simulink model "model5_2022b_localconn"  (R2022b)
settings: Solver=VariableStepAuto  StartTime=0.0  StopTime=10.0  RelTol=1e-3
values from neighbouring files (symbols this model uses):
  eps_local = 50    [init5.m]
  obj1 = [60, 45]    [init5.m]
  obj2 = [30, 25]    [init5.m]
  thr = 5    [init5.m]
undefined symbols (not defined in the file or in its folder): K1, K2, K3, K4, K5, X01, X02, X03, X04, X05, X1d, X1d_dot, X2d, X2d_dot, X3d, X3d_dot, X4d, X4d_dot, X5d, X5d_dot
libraries: slctrlblks x1
settings Model: Creator=dorec  LastModifiedBy=dorec

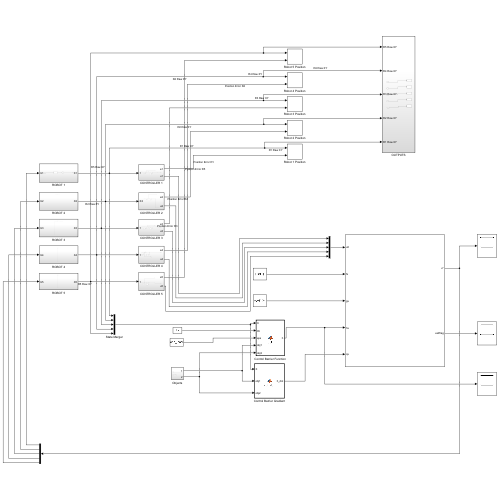
[thumbnail: Simulink's stored preview of the top-level diagram]
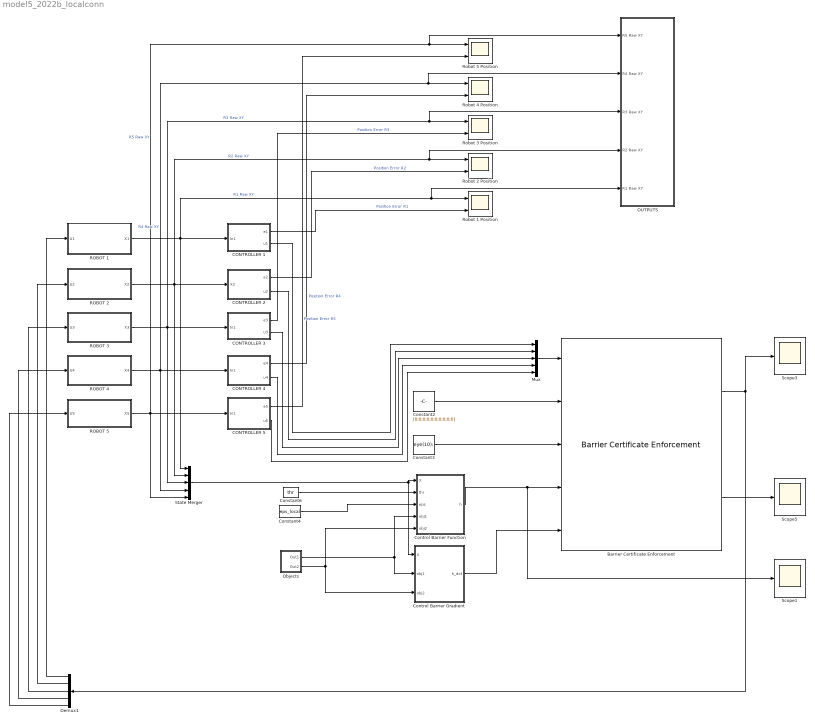
== system model5_2022b_localconn ==
  Barrier Certificate Enforcement : slctrlblks/Barrier Certificate Enforcement  nx=10  nu=10  nc=30  gamma=10  beta=1  external_umax=off  external_umin=off  Ts=0.1  maxiter=200  tol=1e-6  output_exitflag=on
      settings: LibrarySourceBlock=slctrlblks/Constraint Control/Barrier Certificate Enforcement
  CONTROLLER 1 : Subsystem
  CONTROLLER 2 : Subsystem
  CONTROLLER 3 : Subsystem
  CONTROLLER 4 : Subsystem
  CONTROLLER 5 : Subsystem
  Constant2 : Constant  Value=[0;0;0;0;0;0;0;0;0;0]
  Constant3 : Constant  Value=eye(10);
  Constant4 : Constant  Value=eps_local
  Constant6 : Constant  Value=thr
  Control Barrier Function : MATLAB Function  TreatAsAtomicUnit=on
  Control Barrier Gradient : MATLAB Function  TreatAsAtomicUnit=on
  Demux1 : Demux  Outputs=5
  Mux : Mux  Inputs=5
  OUTPUTS : Subsystem
  Objects : Subsystem
  ROBOT 1 : Subsystem
  ROBOT 2 : Subsystem
  ROBOT 3 : Subsystem
  ROBOT 4 : Subsystem
  ROBOT 5 : Subsystem
  Robot 1 Position : Scope  NumInputPorts=2
  Robot 2 Position : Scope  NumInputPorts=2
  Robot 3 Position : Scope  NumInputPorts=2
  Robot 4 Position : Scope  NumInputPorts=2
  Robot 5 Position : Scope  NumInputPorts=2
  Scope1 : Scope
  Scope3 : Scope
  Scope5 : Scope
  State Merger : Mux  Inputs=5
  wires:
  Control Barrier Function/1(h) -> Scope1/1, Barrier Certificate Enforcement/4
  Constant3/1 -> Barrier Certificate Enforcement/3
  Constant2/1 -> Barrier Certificate Enforcement/2
  Barrier Certificate Enforcement/1 -> Scope3/1, Demux1/1
  Mux/1 -> Barrier Certificate Enforcement/1
  Constant6/1 -> Control Barrier Function/2(thr)
  State Merger/1 -> Control Barrier Gradient/1(X), Control Barrier Function/1(X)
  Control Barrier Gradient/1(h_dot) -> Barrier Certificate Enforcement/5
  Barrier Certificate Enforcement/2 -> Scope5/1
  ROBOT 1/1(X1) -> OUTPUTS/5(R1 Raw XY), Robot 1 Position/1, CONTROLLER 1/1(In1), State Merger/1  "R1 Raw XY"
  Demux1/1 -> ROBOT 1/1(U1)
  CONTROLLER 1/2(u1) -> Mux/1
  ROBOT 2/1(X2) -> CONTROLLER 2/1(X2), OUTPUTS/4(R2 Raw XY), Robot 2 Position/1, State Merger/2  "R2 Raw XY"
  Demux1/2 -> ROBOT 2/1(U2)
  CONTROLLER 2/2(u2) -> Mux/2
  ROBOT 3/1(X3) -> OUTPUTS/3(R3 Raw XY), Robot 3 Position/1, CONTROLLER 3/1(In1), State Merger/3  "R3 Raw XY"
  Demux1/3 -> ROBOT 3/1(U3)
  CONTROLLER 3/1(e3) -> Robot 3 Position/2  "Position Error R3"
  CONTROLLER 3/2(u3) -> Mux/3
  ROBOT 4/1(X4) -> CONTROLLER 4/1(In1), OUTPUTS/2(R4 Raw XY), Robot 4 Position/1, State Merger/4  "R4 Raw XY"
  Demux1/4 -> ROBOT 4/1(U4)
  CONTROLLER 4/1(e4) -> Robot 4 Position/2  "Position Error R4"
  CONTROLLER 4/2(u4) -> Mux/4
  ROBOT 5/1(X5) -> OUTPUTS/1(R5 Raw XY), Robot 5 Position/1, CONTROLLER 5/1(In1), State Merger/5  "R5 Raw XY"
  Demux1/5 -> ROBOT 5/1(U5)
  CONTROLLER 5/2(u5) -> Mux/5
  CONTROLLER 5/1(e5) -> Robot 5 Position/2  "Position Error R5"
  CONTROLLER 1/1(e1) -> Robot 1 Position/2  "Position Error R1"
  CONTROLLER 2/1(e2) -> Robot 2 Position/2  "Position Error R2"
  Objects/2(Out2) -> Control Barrier Function/5(obj2), Control Barrier Gradient/3(obj2)
  Objects/1(Out1) -> Control Barrier Function/4(obj1), Control Barrier Gradient/2(obj1)
  Constant4/1 -> Control Barrier Function/3(eps)

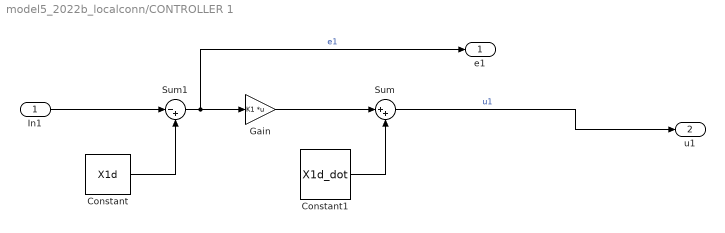
== system model5_2022b_localconn/CONTROLLER 1 ==
  In1 : Inport
  Constant : Constant  Value=X1d
  Constant1 : Constant  Value=X1d_dot
  Gain : Gain  Gain=K1  Multiplication=Matrix(K*u)
  Sum : Sum  Inputs=|++
  Sum1 : Sum  Inputs=|-+
  e1 : Outport
  u1 : Outport  Port=2
  wires:
  Constant/1 -> Sum1/2
  Constant1/1 -> Sum/2
  Sum/1 -> u1/1  "u1"
  Sum1/1 -> e1/1, Gain/1  "e1"
  In1/1 -> Sum1/1
  Gain/1 -> Sum/1

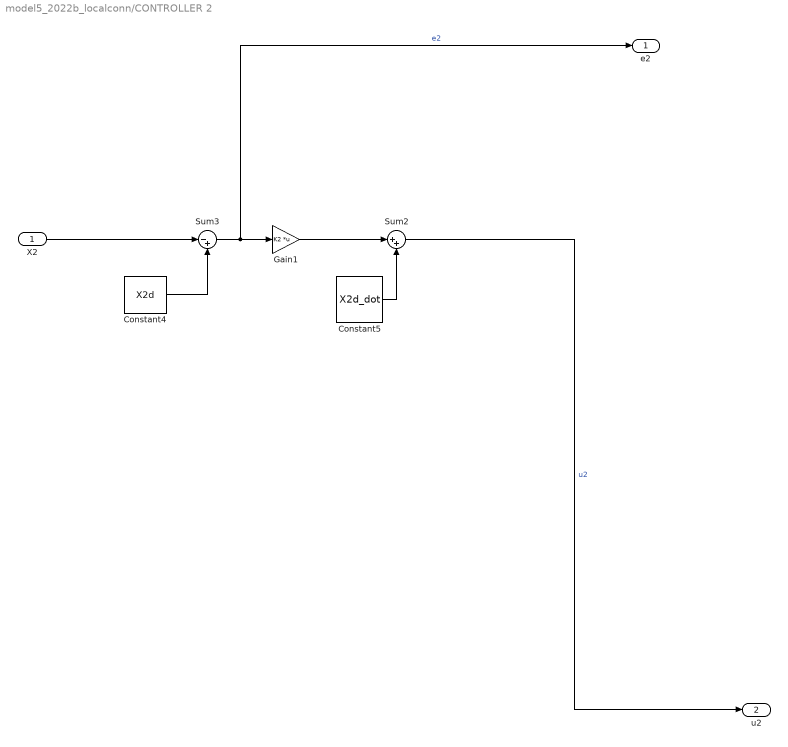
== system model5_2022b_localconn/CONTROLLER 2 ==
  X2 : Inport
  Constant4 : Constant  Value=X2d
  Constant5 : Constant  Value=X2d_dot
  Gain1 : Gain  Gain=K2  Multiplication=Matrix(K*u)
  Sum2 : Sum  Inputs=|++
  Sum3 : Sum  Inputs=|-+
  e2 : Outport
  u2 : Outport  Port=2
  wires:
  Constant4/1 -> Sum3/2
  Constant5/1 -> Sum2/2
  Sum3/1 -> e2/1, Gain1/1  "e2"
  Gain1/1 -> Sum2/1
  Sum2/1 -> u2/1  "u2"
  X2/1 -> Sum3/1

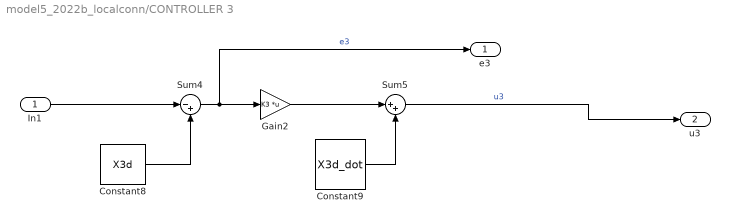
== system model5_2022b_localconn/CONTROLLER 3 ==
  In1 : Inport
  Constant8 : Constant  Value=X3d
  Constant9 : Constant  Value=X3d_dot
  Gain2 : Gain  Gain=K3  Multiplication=Matrix(K*u)
  Sum4 : Sum  Inputs=|-+
  Sum5 : Sum  Inputs=|++
  e3 : Outport
  u3 : Outport  Port=2
  wires:
  Constant9/1 -> Sum5/2
  Gain2/1 -> Sum5/1
  Sum4/1 -> e3/1, Gain2/1  "e3"
  Constant8/1 -> Sum4/2
  Sum5/1 -> u3/1  "u3"
  In1/1 -> Sum4/1

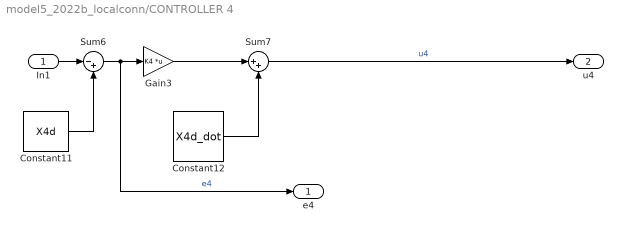
== system model5_2022b_localconn/CONTROLLER 4 ==
  In1 : Inport
  Constant11 : Constant  Value=X4d
  Constant12 : Constant  Value=X4d_dot
  Gain3 : Gain  Gain=K4  Multiplication=Matrix(K*u)
  Sum6 : Sum  Inputs=|-+
  Sum7 : Sum  Inputs=|++
  e4 : Outport
  u4 : Outport  Port=2
  wires:
  Sum6/1 -> e4/1, Gain3/1  "e4"
  Gain3/1 -> Sum7/1
  Constant11/1 -> Sum6/2
  Constant12/1 -> Sum7/2
  Sum7/1 -> u4/1  "u4"
  In1/1 -> Sum6/1

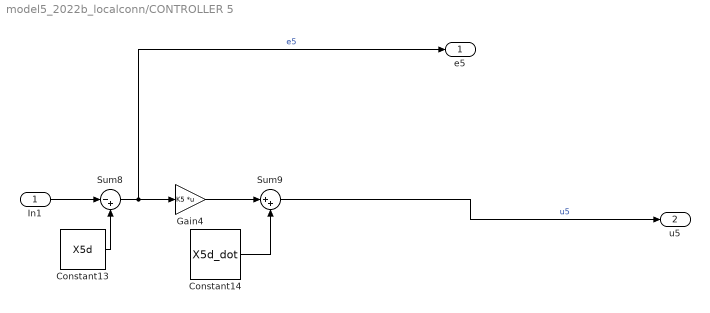
== system model5_2022b_localconn/CONTROLLER 5 ==
  In1 : Inport
  Constant13 : Constant  Value=X5d
  Constant14 : Constant  Value=X5d_dot
  Gain4 : Gain  Gain=K5  Multiplication=Matrix(K*u)
  Sum8 : Sum  Inputs=|-+
  Sum9 : Sum  Inputs=|++
  e5 : Outport
  u5 : Outport  Port=2
  wires:
  Sum8/1 -> e5/1, Gain4/1  "e5"
  Constant13/1 -> Sum8/2
  Gain4/1 -> Sum9/1
  In1/1 -> Sum8/1
  Constant14/1 -> Sum9/2
  Sum9/1 -> u5/1  "u5"

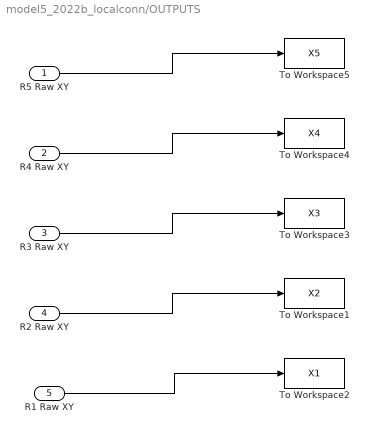
== system model5_2022b_localconn/OUTPUTS ==
  R5 Raw XY : Inport
  R4 Raw XY : Inport  Port=2
  R3 Raw XY : Inport  Port=3
  R2 Raw XY : Inport  Port=4
  R1 Raw XY : Inport  Port=5
  To Workspace1 : ToWorkspace  VariableName=X2  SaveFormat=Timeseries  SampleTime=-1
  To Workspace2 : ToWorkspace  VariableName=X1  SaveFormat=Timeseries  SampleTime=-1
  To Workspace3 : ToWorkspace  VariableName=X3  SaveFormat=Timeseries  SampleTime=-1
  To Workspace4 : ToWorkspace  VariableName=X4  SaveFormat=Timeseries  SampleTime=-1
  To Workspace5 : ToWorkspace  VariableName=X5  SaveFormat=Timeseries  SampleTime=-1
  wires:
  R5 Raw XY/1 -> To Workspace5/1
  R2 Raw XY/1 -> To Workspace1/1
  R1 Raw XY/1 -> To Workspace2/1
  R3 Raw XY/1 -> To Workspace3/1
  R4 Raw XY/1 -> To Workspace4/1

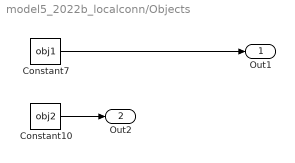
== system model5_2022b_localconn/Objects ==
  Constant10 : Constant  Value=obj2
  Constant7 : Constant  Value=obj1
  Out1 : Outport
  Out2 : Outport  Port=2
  wires:
  Constant10/1 -> Out2/1
  Constant7/1 -> Out1/1

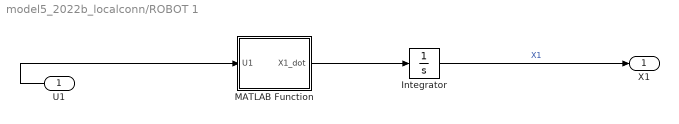
== system model5_2022b_localconn/ROBOT 1 ==
  U1 : Inport
  Integrator : Integrator  InitialCondition=X01
  MATLAB Function : MATLAB Function  TreatAsAtomicUnit=on
  X1 : Outport
  wires:
  MATLAB Function/1(X1_dot) -> Integrator/1
  Integrator/1 -> X1/1  "X1"
  U1/1 -> MATLAB Function/1(U1)

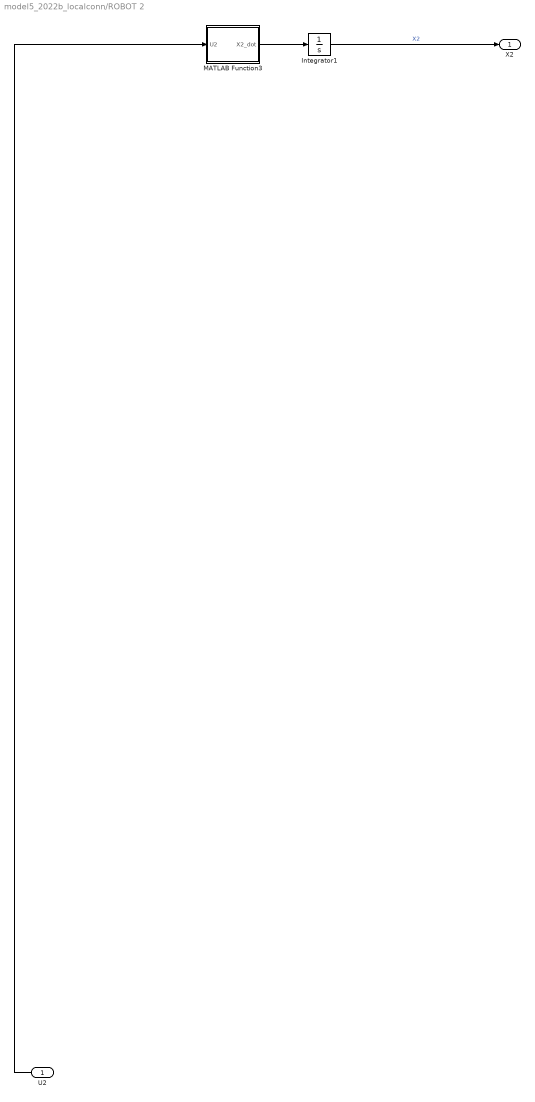
== system model5_2022b_localconn/ROBOT 2 ==
  U2 : Inport
  Integrator1 : Integrator  InitialCondition=X02
  MATLAB Function3 : MATLAB Function  TreatAsAtomicUnit=on
  X2 : Outport
  wires:
  MATLAB Function3/1(X2_dot) -> Integrator1/1
  U2/1 -> MATLAB Function3/1(U2)
  Integrator1/1 -> X2/1  "X2"

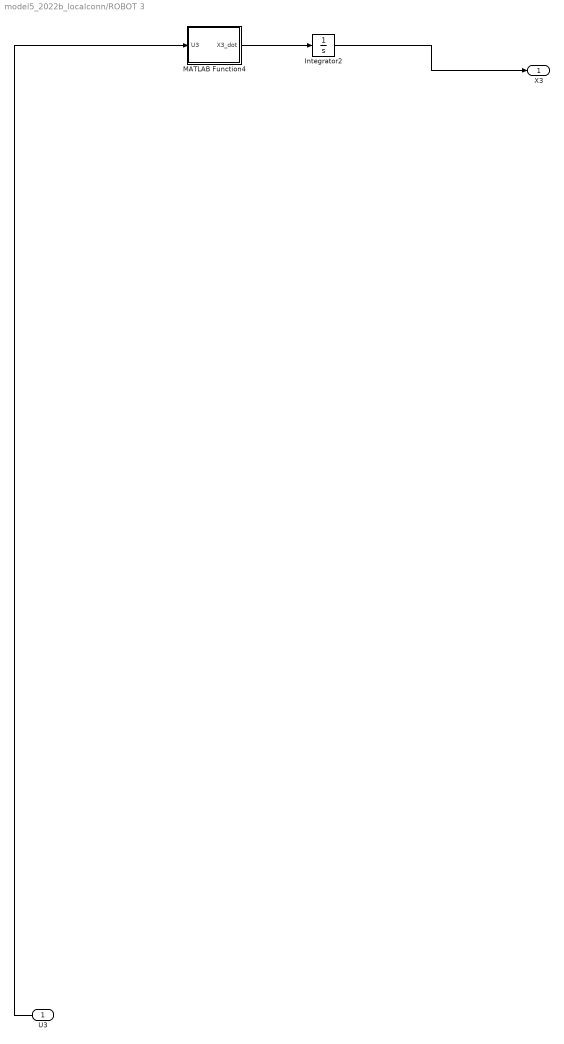
== system model5_2022b_localconn/ROBOT 3 ==
  U3 : Inport
  Integrator2 : Integrator  InitialCondition=X03
  MATLAB Function4 : MATLAB Function  TreatAsAtomicUnit=on
  X3 : Outport
  wires:
  U3/1 -> MATLAB Function4/1(U3)
  MATLAB Function4/1(X3_dot) -> Integrator2/1
  Integrator2/1 -> X3/1

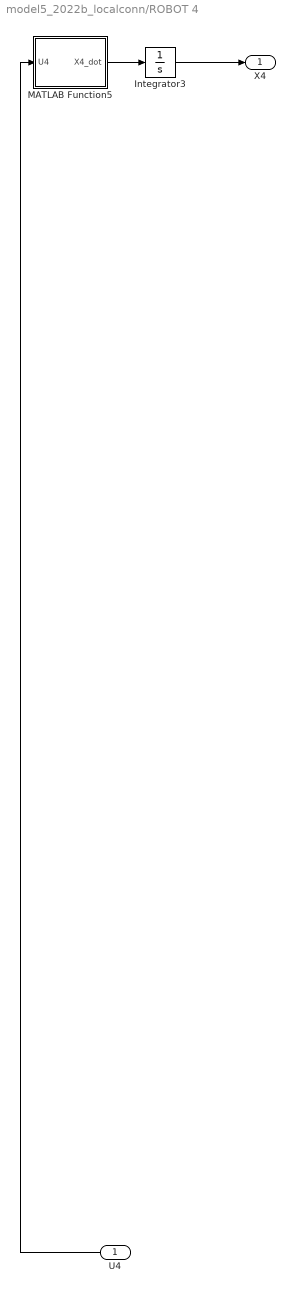
== system model5_2022b_localconn/ROBOT 4 ==
  U4 : Inport
  Integrator3 : Integrator  InitialCondition=X04
  MATLAB Function5 : MATLAB Function  TreatAsAtomicUnit=on
  X4 : Outport
  wires:
  MATLAB Function5/1(X4_dot) -> Integrator3/1
  U4/1 -> MATLAB Function5/1(U4)
  Integrator3/1 -> X4/1

== system model5_2022b_localconn/ROBOT 5 ==
  U5 : Inport
  Integrator4 : Integrator  InitialCondition=X05
  MATLAB Function6 : MATLAB Function  TreatAsAtomicUnit=on
  X5 : Outport
  wires:
  U5/1 -> MATLAB Function6/1(U5)
  MATLAB Function6/1(X5_dot) -> Integrator4/1
  Integrator4/1 -> X5/1

== matlab function model5_2022b_localconn/Control Barrier Function ==
  data: X input; thr input; eps input; h output; obj1 input; obj2 input
function h = cbf(X, thr, eps, obj1, obj2)

    %RESHAPES the vector from the mux (not stacked)
    Nvectors=numel(X)/2;
    X=reshape(X,2,Nvectors);
    
    %Extracts components col by col
    X1 = X(:,1);  
    X2 = X(:,2); 
    X3 = X(:,3);  
    X4 = X(:,4);  
    X5 = X(:,5);  

    h12 = norm(X1 - X2) - thr;
    h13 = norm(X1 - X3) - thr;
    h14 = norm(X1 - X4) - thr;
    h15 = norm(X1 - X5) - thr;

    h23 = norm(X2 - X3) - thr;
    h24 = norm(X2 - X4) - thr;
    h25 = norm(X2 - X5) - thr;

    h34 = norm(X3 - X4) - thr;
    h35 = norm(X3 - X5) - thr;

    h45 = norm(X4 - X5) - thr;


    h1o1 = norm(X1 - obj1) - thr;
    h2o1 = norm(X2 - obj1) - thr;
    h3o1 = norm(X3 - obj1) - thr;
    h4o1 = norm(X4 - obj1) - thr;
    h5o1 = norm(X5 - obj1) - thr;

    h1o2 = norm(X1 - obj2) - thr;
    h2o2 = norm(X2 - obj2) - thr;
    h3o2 = norm(X3 - obj2) - thr;
    h4o2 = norm(X4 - obj2) - thr;
    h5o2 = norm(X5 - obj2) - thr;

    hc12 = eps - norm(X1 - X2);
    hc13 = eps - norm(X1 - X3);
    hc14 = eps - norm(X1 - X4);
    hc15 = eps - norm(X1 - X5);

    hc23 = eps - norm(X2 - X3);
    hc24 = eps - norm(X2 - X4);
    hc25 = eps - norm(X2 - X5);

    hc34 = eps - norm(X3 - X4);
    hc35 = eps - norm(X3 - X5);

    hc45 = eps - norm(X4 - X5);


    h = [ h12; h13; h14; h15;
          h23; h24; h25;
          h34; h35;
          h45;
          h1o1; h2o1; h3o1; h4o1; h5o1;
          h1o2; h2o2; h3o2; h4o2; h5o2;
          hc12; hc13; hc14; hc15;
          hc23; hc24; hc25;
          hc34; hc35;
          hc45;];
end

== matlab function model5_2022b_localconn/ROBOT 1/MATLAB Function ==
  data: U1 input size=[2 1]; X1_dot output
function X1_dot = dynamics(U1)

x1_dot = U1(1);
y1_dot = U1(2);

X1_dot = [x1_dot; y1_dot];

== matlab function model5_2022b_localconn/Control Barrier Gradient ==
  data: X input; obj1 input; h_dot output; obj2 input
function h_dot = cbf_dot(X, obj1, obj2)
    %RESHAPES the vector from the mux (not stacked)
    Nvectors=numel(X)/2;
    X=reshape(X,2,Nvectors);
    
    %Extracts components col by col
    X1 = X(:,1);  
    X2 = X(:,2); 
    X3 = X(:,3);  
    X4 = X(:,4);  
    X5 = X(:,5);  

    n12 = (X1 - X2)/norm(X1 - X2);
    n13 = (X1 - X3)/norm(X1 - X3);
    n14 = (X1 - X4)/norm(X1 - X4);
    n15 = (X1 - X5)/norm(X1 - X5);

    n23 = (X2 - X3)/norm(X2 - X3);
    n24 = (X2 - X4)/norm(X2 - X4);
    n25 = (X2 - X5)/norm(X2 - X5);

    n34 = (X3 - X4)/norm(X3 - X4);
    n35 = (X3 - X5)/norm(X3 - X5);

    n45 = (X4 - X5)/norm(X4 - X5);

    
    n1o1 = (X1 - obj1)/norm(X1 - obj1);
    n2o1 = (X2 - obj1)/norm(X2 - obj1);
    n3o1 = (X3 - obj1)/norm(X3 - obj1);
    n4o1 = (X4 - obj1)/norm(X4 - obj1);
    n5o1 = (X5 - obj1)/norm(X5 - obj1);

    
    n1o2 = (X1 - obj2)/norm(X1 - obj2);
    n2o2 = (X2 - obj2)/norm(X2 - obj2);
    n3o2 = (X3 - obj2)/norm(X3 - obj2);
    n4o2 = (X4 - obj2)/norm(X4 - obj2);
    n5o2 = (X5 - obj2)/norm(X5 - obj2);

    nc12 = -n12;
    nc13 = -n13;
    nc14 = -n14;
    nc15 = -n15;
    
    nc23 = -n23;
    nc24 = -n24;
    nc25 = -n25;

    nc34 = -n34;
    nc35 = -n35;

    nc45 = -n45;

    h_dot = [
        
        n12(1) n12(2)  -n12(1) -n12(2)   0 0   0 0   0 0; 
        n13(1) n13(2)   0 0  -n13(1) -n13(2)  0 0   0 0; 
        n14(1) n14(2)   0 0   0 0  -n14(1) -n14(2)  0 0; 
        n15(1) n15(2)   0 0   0 0   0 0  -n15(1) -n15(2); 

        0 0  n23(1) n23(2)  -n23(1) -n23(2)  0 0   0 0; 
        0 0  n24(1) n24(2)   0 0  -n24(1) -n24(2)  0 0; 
        0 0  n25(1) n25(2)   0 0   0 0  -n25(1) -n25(2); 

        0 0   0 0  n34(1) n34(2)  -n34(1) -n34(2)  0 0; 
        0 0   0 0  n35(1) n35(2)   0 0  -n35(1) -n35(2); 

        0 0   0 0   0 0  n45(1) n45(2)  -n45(1) -n45(2); 

        n1o1(1) n1o1(2)  0 0 0 0 0 0 0 0; 
        0 0  n2o1(1) n2o1(2)  0 0 0 0 0 0; 
        0 0  0 0  n3o1(1) n3o1(2)  0 0 0 0; 
        0 0  0 0  0 0  n4o1(1) n4o1(2)  0 0; 
        0 0  0 0  0 0  0 0  n5o1(1) n5o1(2); 

        n1o2(1) n1o2(2)  0 0 0 0 0 0 0 0;
        0 0  n2o2(1) n2o2(2)  0 0 0 0 0 0; 
        0 0  0 0  n3o2(1) n3o2(2)  0 0 0 0;
        0 0  0 0  0 0  n4o2(1) n4o2(2)  0 0;
        0 0  0 0  0 0  0 0  n5o2(1) n5o2(2);

        nc12(1) nc12(2)  -nc12(1) -nc12(2)   0 0   0 0   0 0; 
        nc13(1) nc13(2)   0 0  -nc13(1) -nc13(2)  0 0   0 0; 
        nc14(1) nc14(2)   0 0   0 0  -nc14(1) -nc14(2)  0 0; 
        nc15(1) nc15(2)   0 0   0 0   0 0  -nc15(1) -nc15(2); 

        0 0  nc23(1) nc23(2)  -nc23(1) -nc23(2)  0 0   0 0; 
        0 0  nc24(1) nc24(2)   0 0  -nc24(1) -nc24(2)  0 0; 
        0 0  nc25(1) nc25(2)   0 0   0 0  -nc25(1) -nc25(2); 

        0 0   0 0  nc34(1) nc34(2)  -nc34(1) -nc34(2)  0 0; 
        0 0   0 0  nc35(1) nc35(2)   0 0  -nc35(1) -nc35(2); 

        0 0   0 0   0 0  nc45(1) nc45(2)  -nc45(1) -nc45(2); 

    ];
end

== matlab function model5_2022b_localconn/ROBOT 2/MATLAB Function3 ==
  data: U2 input size=[2 1]; X2_dot output
function X2_dot = dynamics(U2)

x2_dot = U2(1);
y2_dot = U2(2);

X2_dot = [x2_dot; y2_dot];

== matlab function model5_2022b_localconn/ROBOT 3/MATLAB Function4 ==
  data: U3 input size=[2 1]; X3_dot output
function X3_dot = dynamics(U3)

x3_dot = U3(1);
y3_dot = U3(2);

X3_dot = [x3_dot; y3_dot];

== matlab function model5_2022b_localconn/ROBOT 4/MATLAB Function5 ==
  data: U4 input size=[2 1]; X4_dot output
function X4_dot = dynamics(U4)

x4_dot = U4(1);
y4_dot = U4(2);

X4_dot = [x4_dot; y4_dot];

== matlab function model5_2022b_localconn/ROBOT 5/MATLAB Function6 ==
  data: U5 input size=[2 1]; X5_dot output
function X5_dot = dynamics(U5)

x5_dot = U5(1);
y5_dot = U5(2);

X5_dot = [x5_dot; y5_dot];
